simulink model "q10"  (R2022b)
settings: Solver=VariableStepAuto  StartTime=0.0  StopTime=10.0  RelTol=1e-3
settings Model: Creator=asus  LastModifiedBy=asus

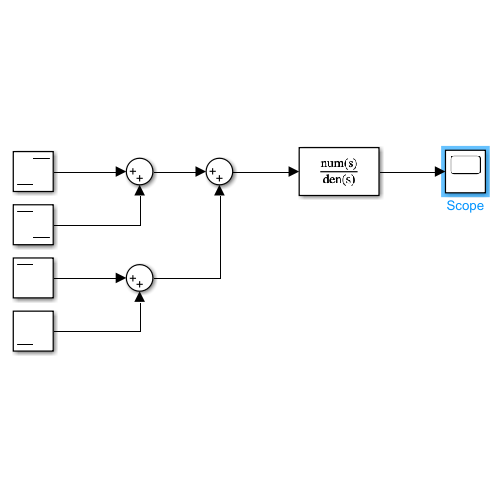
[thumbnail: Simulink's stored preview of the top-level diagram]
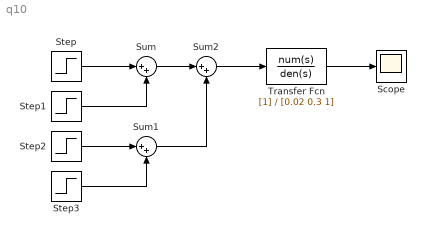
== system q10 ==
  Scope : Scope
  Step : Step  Time=2  SampleTime=0
  Step1 : Step  Time=4  After=-1  SampleTime=0
  Step2 : Step  Time=6  After=-1  SampleTime=0
  Step3 : Step  Time=8  SampleTime=0
  Sum : Sum  Inputs=|++
  Sum1 : Sum  Inputs=|++
  Sum2 : Sum  Inputs=|++
  Transfer Fcn : TransferFcn  Denominator=[0.02 0.3 1]
  wires:
  Step/1 -> Sum/1
  Step1/1 -> Sum/2
  Sum/1 -> Sum2/1
  Step2/1 -> Sum1/1
  Step3/1 -> Sum1/2
  Sum1/1 -> Sum2/2
  Sum2/1 -> Transfer Fcn/1
  Transfer Fcn/1 -> Scope/1
